simulink model "power_system"  (R2019a)
settings: Solver=FixedStepAuto  StartTime=0.0  StopTime=10.0  RelTol=1e-3
values from neighbouring files (symbols this model uses):
  numberOfBuses = 2    [init.m]
  numberOfGenerators = 4    [init.m]
undefined symbols (not defined in the file or in its folder): magnitude
libraries: simulink x8
(part 2 of 2)

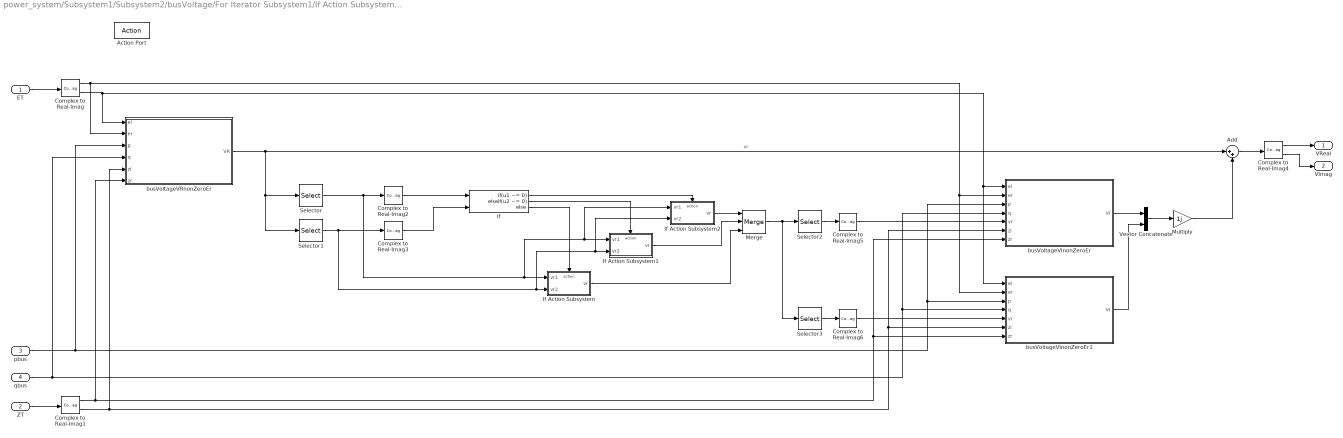
== system power_system/Subsystem1/Subsystem2/busVoltage/For Iterator Subsystem1/If Action Subsystem1/If Action Subsystem1 ==
  ET : Inport
  ZT : Inport  Port=2
  pbus : Inport  Port=3
  qbus : Inport  Port=4
  Action Port : ActionPort  ActionPortLabel=elseif(u1>u2)
  Add : Sum  Inputs=|++
  Complex to Real-Imag : ComplexToRealImag
  Complex to Real-Imag1 : ComplexToRealImag
  Complex to Real-Imag2 : ComplexToRealImag  Output=Imag
  Complex to Real-Imag3 : ComplexToRealImag  Output=Imag
  Complex to Real-Imag4 : ComplexToRealImag
  Complex to Real-Imag5 : ComplexToRealImag  Output=Real
  Complex to Real-Imag6 : ComplexToRealImag  Output=Real
  If : If  NumInputs=2  IfExpression=u1 ~= 0  ElseIfExpressions=u2 ~= 0
  If Action Subsystem : Subsystem  TreatAsAtomicUnit=on
  If Action Subsystem1 : Subsystem  TreatAsAtomicUnit=on
  If Action Subsystem2 : Subsystem  TreatAsAtomicUnit=on
  Merge : Merge  Inputs=3
  Multiply : Gain  Gain=1j
  Selector : Selector  InputPortWidth=2  IndexOptions=Index vector (dialog)  Indices=[1]  OutputSizes=1
  Selector1 : Selector  InputPortWidth=2  IndexOptions=Index vector (dialog)  Indices=[2]  OutputSizes=1
  Selector2 : Selector  InputPortWidth=2  IndexOptions=Index vector (dialog)  Indices=1  OutputSizes=1
  Selector3 : Selector  InputPortWidth=2  IndexOptions=Index vector (dialog)  Indices=2  OutputSizes=1
  Vector Concatenate : Concatenate
  busVoltageVInonZeroEr : Subsystem
  busVoltageVInonZeroEr1 : Subsystem
  busVoltageVRnonZeroEr : Subsystem
  VReal : Outport
  VImag : Outport  Port=2
  wires:
  Add/1 -> Complex to Real-Imag4/1
  Multiply/1 -> Add/2
  Vector Concatenate/1 -> Multiply/1
  busVoltageVInonZeroEr1/1(VI) -> Vector Concatenate/2
  busVoltageVInonZeroEr/1(VI) -> Vector Concatenate/1
  Complex to Real-Imag1/1 -> busVoltageVRnonZeroEr/6(zr), busVoltageVInonZeroEr1/7(zr), busVoltageVInonZeroEr/7(zr)
  Complex to Real-Imag1/2 -> busVoltageVRnonZeroEr/5(zi), busVoltageVInonZeroEr1/6(zi), busVoltageVInonZeroEr/6(zi)
  qbus/1 -> busVoltageVInonZeroEr1/4(q), busVoltageVInonZeroEr/4(q), busVoltageVRnonZeroEr/4(q)
  pbus/1 -> busVoltageVRnonZeroEr/3(p), busVoltageVInonZeroEr1/3(p), busVoltageVInonZeroEr/3(p)
  Complex to Real-Imag/1 -> busVoltageVRnonZeroEr/2(er), busVoltageVInonZeroEr1/2(er), busVoltageVInonZeroEr/2(er)
  Complex to Real-Imag/2 -> busVoltageVRnonZeroEr/1(ei), busVoltageVInonZeroEr1/1(ei), busVoltageVInonZeroEr/1(ei)
  Selector2/1 -> Complex to Real-Imag5/1
  Selector3/1 -> Complex to Real-Imag6/1
  Merge/1 -> Selector3/1, Selector2/1
  If Action Subsystem/1(vr) -> Merge/3
  If Action Subsystem1/1(vr) -> Merge/2
  If Action Subsystem2/1(vr) -> Merge/1
  Selector1/1 -> Complex to Real-Imag3/1, If Action Subsystem1/2(vr2), If Action Subsystem2/2(vr2), If Action Subsystem/2(vr2)
  If/3 -> If Action Subsystem/Action
  If/2 -> If Action Subsystem1/Action
  If/1 -> If Action Subsystem2/Action
  Complex to Real-Imag3/1 -> If/2
  Complex to Real-Imag2/1 -> If/1
  Selector/1 -> Complex to Real-Imag2/1, If Action Subsystem1/1(vr1), If Action Subsystem2/1(vr1), If Action Subsystem/1(vr1)
  busVoltageVRnonZeroEr/1(VR) -> Add/1, Selector/1, Selector1/1  "vr"
  ZT/1 -> Complex to Real-Imag1/1
  ET/1 -> Complex to Real-Imag/1
  Complex to Real-Imag4/2 -> VImag/1
  Complex to Real-Imag4/1 -> VReal/1
  Complex to Real-Imag5/1 -> busVoltageVInonZeroEr/5(vr)
  Complex to Real-Imag6/1 -> busVoltageVInonZeroEr1/5(vr)

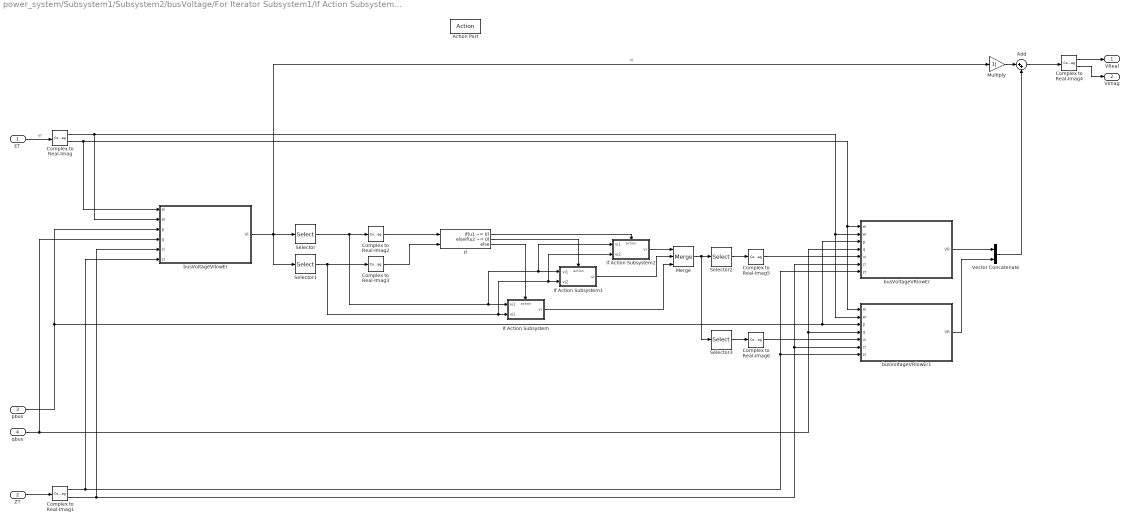
== system power_system/Subsystem1/Subsystem2/busVoltage/For Iterator Subsystem1/If Action Subsystem1/If Action Subsystem2 ==
  ET : Inport
  ZT : Inport  Port=2
  pbus : Inport  Port=3
  qbus : Inport  Port=4
  Action Port : ActionPort  ActionPortLabel=else
  Add : Sum  Inputs=|++
  Complex to Real-Imag : ComplexToRealImag
  Complex to Real-Imag1 : ComplexToRealImag
  Complex to Real-Imag2 : ComplexToRealImag  Output=Imag
  Complex to Real-Imag3 : ComplexToRealImag  Output=Imag
  Complex to Real-Imag4 : ComplexToRealImag
  Complex to Real-Imag5 : ComplexToRealImag  Output=Real
  Complex to Real-Imag6 : ComplexToRealImag  Output=Real
  If : If  NumInputs=2  IfExpression=u1 ~= 0  ElseIfExpressions=u2 ~= 0
  If Action Subsystem : Subsystem  TreatAsAtomicUnit=on
  If Action Subsystem1 : Subsystem  TreatAsAtomicUnit=on
  If Action Subsystem2 : Subsystem  TreatAsAtomicUnit=on
  Merge : Merge  Inputs=3
  Multiply : Gain  Gain=1j
  Selector : Selector  InputPortWidth=2  IndexOptions=Index vector (dialog)  Indices=[1]  OutputSizes=1
  Selector1 : Selector  InputPortWidth=2  IndexOptions=Index vector (dialog)  Indices=[2]  OutputSizes=1
  Selector2 : Selector  InputPortWidth=2  IndexOptions=Index vector (dialog)  Indices=[1]  OutputSizes=1
  Selector3 : Selector  InputPortWidth=2  IndexOptions=Index vector (dialog)  Indices=[2]  OutputSizes=1
  Vector Concatenate : Concatenate
  busVoltageVIlowEr : Subsystem
  busVoltageVRlowEr : Subsystem
  busVoltageVRlowEr1 : Subsystem
  VReal : Outport
  VImag : Outport  Port=2
  wires:
  Vector Concatenate/1 -> Add/2
  Multiply/1 -> Add/1
  Selector3/1 -> Complex to Real-Imag6/1
  Selector2/1 -> Complex to Real-Imag5/1
  ET/1 -> Complex to Real-Imag/1  "vr"
  busVoltageVRlowEr1/1(VR) -> Vector Concatenate/2
  busVoltageVRlowEr/1(VR) -> Vector Concatenate/1
  If/3 -> If Action Subsystem/Action
  Selector1/1 -> Complex to Real-Imag3/1, If Action Subsystem/2(vi2), If Action Subsystem1/2(vi2), If Action Subsystem2/2(vi2)
  If Action Subsystem1/1(vi) -> Merge/2
  If Action Subsystem2/1(vi) -> Merge/1
  Selector/1 -> Complex to Real-Imag2/1, If Action Subsystem/1(vi1), If Action Subsystem1/1(vi1), If Action Subsystem2/1(vi1)
  If Action Subsystem/1(vi) -> Merge/3
  If/2 -> If Action Subsystem1/Action
  Merge/1 -> Selector3/1, Selector2/1
  If/1 -> If Action Subsystem2/Action
  Complex to Real-Imag2/1 -> If/1
  Complex to Real-Imag3/1 -> If/2
  busVoltageVIlowEr/1(VI) -> Selector1/1, Multiply/1, Selector/1  "vi"
  qbus/1 -> busVoltageVIlowEr/4(q), busVoltageVRlowEr/4(q), busVoltageVRlowEr1/4(q)
  pbus/1 -> busVoltageVRlowEr/3(p), busVoltageVRlowEr1/3(p), busVoltageVIlowEr/3(p)
  Complex to Real-Imag/2 -> busVoltageVRlowEr/1(ei), busVoltageVRlowEr1/1(ei), busVoltageVIlowEr/1(ei)
  Complex to Real-Imag/1 -> busVoltageVRlowEr/2(er), busVoltageVRlowEr1/2(er), busVoltageVIlowEr/2(er)
  Complex to Real-Imag1/1 -> busVoltageVRlowEr/7(zr), busVoltageVRlowEr1/7(zr), busVoltageVIlowEr/6(zr)
  Complex to Real-Imag1/2 -> busVoltageVIlowEr/5(zi), busVoltageVRlowEr/6(zi), busVoltageVRlowEr1/6(zi)
  ZT/1 -> Complex to Real-Imag1/1
  Complex to Real-Imag4/1 -> VReal/1
  Complex to Real-Imag4/2 -> VImag/1
  Add/1 -> Complex to Real-Imag4/1
  Complex to Real-Imag5/1 -> busVoltageVRlowEr/5(vi)
  Complex to Real-Imag6/1 -> busVoltageVRlowEr1/5(vi)

== system power_system/Subsystem1/Subsystem2/busVoltage/For Iterator Subsystem1/If Action Subsystem1/If Action Subsystem3 ==
  Action Port : ActionPort  ActionPortLabel=if(u1 < u2)
  Constant : Constant
  v : Outport
  wires:
  Constant/1 -> v/1

== system power_system/Subsystem1/Subsystem2/busVoltage/For Iterator Subsystem1/If Action Subsystem1/If Action Subsystem4 ==
  Action Port : ActionPort  ActionPortLabel=else
  Constant : Constant  Value=2
  v : Outport
  wires:
  Constant/1 -> v/1

== system power_system/Subsystem1/Subsystem2/busVoltage/For Iterator Subsystem1/If Action Subsystem1/map to [-pi, pi] ==
  u : Inport
  Add : Sum  Inputs=||+-+
  Compare To Constant : simulink/Logic and Bit Operations/Compare To Constant  relop=>  const=pi  OutDataTypeStr=boolean
  Compare To Constant1 : simulink/Logic and Bit Operations/Compare To Constant  relop=<  const=-pi  OutDataTypeStr=boolean
  Constant : Constant  Value=2*pi
  Gain1 : Gain  Gain=2*pi
  Gain2 : Gain  Gain=2*pi
  Mod : Math  Operator=mod  SaturateOnIntegerOverflow=on
  y : Outport
  wires:
  Compare To Constant1/1 -> Gain2/1
  Compare To Constant/1 -> Gain1/1
  u/1 -> Mod/1
  Gain1/1 -> Add/2
  Mod/1 -> Compare To Constant/1, Compare To Constant1/1, Add/1
  Add/1 -> y/1
  Constant/1 -> Mod/2
  Gain2/1 -> Add/3

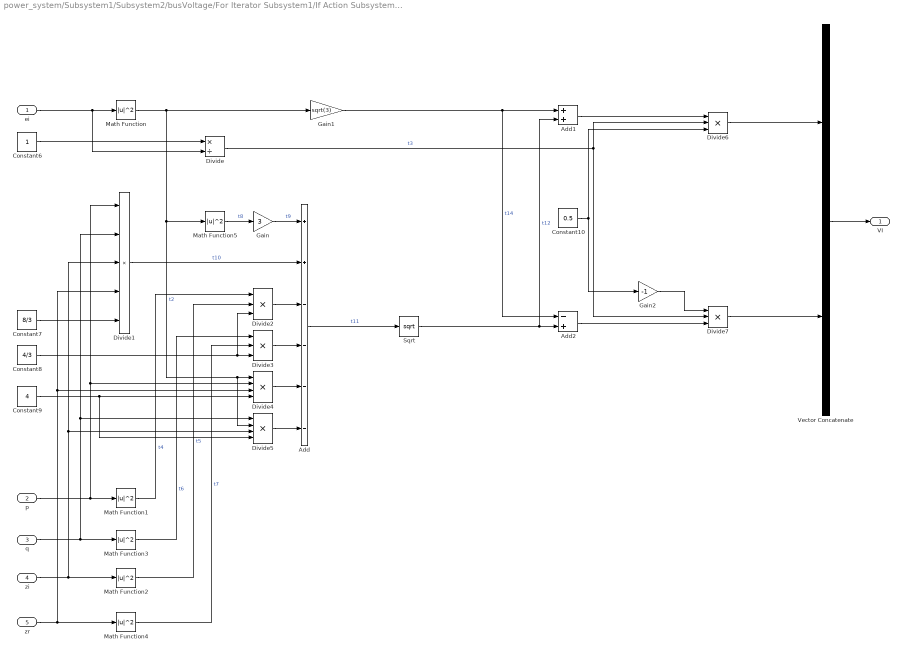
== system power_system/Subsystem1/Subsystem2/busVoltage/For Iterator Subsystem1/If Action Subsystem1/If Action Subsystem/busVoltageVIzeroEr ==
  ei : Inport
  p : Inport  Port=2
  q : Inport  Port=3
  zi : Inport  Port=4
  zr : Inport  Port=5
  Add : Sum  Inputs=++----
  Add1 : Sum
  Add2 : Sum  Inputs=-+
  Constant10 : Constant  Value=0.5
  Constant6 : Constant
  Constant7 : Constant  Value=8/3
  Constant8 : Constant  Value=4/3
  Constant9 : Constant  Value=4
  Divide : Product  Inputs=*/
  Divide1 : Product  Inputs=5
  Divide{2..3,6..7} (4 alike) : Product  Inputs=3
  Divide4 : Product  Inputs=4
  Divide5 : Product  Inputs=4
  Gain : Gain  Gain=3
  Gain1 : Gain  Gain=sqrt(3)
  Gain2 : Gain  Gain=-1
  Math Function{,1..5} (6 alike) : Math  Operator=magnitude^2  SaturateOnIntegerOverflow=on
  Sqrt : Sqrt  SaturateOnIntegerOverflow=on
  Vector Concatenate : Concatenate
  VI : Outport
  wires:
  Math Function1/1 -> Divide2/1  "t4"
  Add2/1 -> Divide7/3
  Gain2/1 -> Divide7/1
  Divide2/1 -> Add/3
  Divide1/1 -> Add/2  "t10"
  Divide6/1 -> Vector Concatenate/1
  Math Function3/1 -> Divide3/1  "t6"
  Math Function5/1 -> Gain/1  "t8"
  Constant6/1 -> Divide/1
  Add/1 -> Sqrt/1  "t11"
  Sqrt/1 -> Add2/2, Add1/2  "t12"
  zr/1 -> Math Function4/1, Divide1/4, Divide4/3
  Gain/1 -> Add/1  "t9"
  Add1/1 -> Divide6/1
  Divide/1 -> Divide7/2, Divide6/2  "t3"
  Gain1/1 -> Add1/1, Add2/1  "t14"
  Constant10/1 -> Gain2/1, Divide6/3
  p/1 -> Math Function1/1, Divide1/1, Divide4/2
  Math Function/1 -> Gain1/1, Divide4/1, Divide5/2, Math Function5/1  "t2"
  Constant9/1 -> Divide4/4, Divide5/4
  Constant8/1 -> Divide2/3, Divide3/3
  ei/1 -> Math Function/1, Divide/2
  Math Function2/1 -> Divide2/2  "t5"
  Vector Concatenate/1 -> VI/1
  Constant7/1 -> Divide1/5
  Divide7/1 -> Vector Concatenate/2
  q/1 -> Math Function3/1, Divide1/2, Divide5/1
  Divide4/1 -> Add/5
  Math Function4/1 -> Divide3/2  "t7"
  Divide5/1 -> Add/6
  zi/1 -> Math Function2/1, Divide1/3, Divide5/3
  Divide3/1 -> Add/4

== system power_system/Subsystem1/Subsystem2/busVoltage/For Iterator Subsystem1/If Action Subsystem1/If Action Subsystem/busVoltageVRzeroEr ==
  ei : Inport
  p : Inport  Port=2
  q : Inport  Port=3
  zi : Inport  Port=4
  zr : Inport  Port=5
  Add : Sum  Inputs=|+-
  Divide : Product
  Divide1 : Product
  Divide2 : Product  Inputs=/*
  Gain : Gain  Gain=sqrt(3)/3
  VR : Outport
  wires:
  Divide1/1 -> Add/1
  Divide/1 -> Add/2
  zi/1 -> Divide1/2
  Divide2/1 -> VR/1
  ei/1 -> Divide2/1
  q/1 -> Divide/1
  Add/1 -> Gain/1
  zr/1 -> Divide/2
  p/1 -> Divide1/1
  Gain/1 -> Divide2/2

== system power_system/Subsystem1/Subsystem2/busVoltage/For Iterator Subsystem1/If Action Subsystem1/If Action Subsystem1/If Action Subsystem ==
  vr1 : Inport
  vr2 : Inport  Port=2
  Action Port : ActionPort  ActionPortLabel=else
  Vector Concatenate : Concatenate
  vr : Outport
  wires:
  Vector Concatenate/1 -> vr/1
  vr2/1 -> Vector Concatenate/2
  vr1/1 -> Vector Concatenate/1

== system power_system/Subsystem1/Subsystem2/busVoltage/For Iterator Subsystem1/If Action Subsystem1/If Action Subsystem1/If Action Subsystem1 ==
  vr1 : Inport
  vr2 : Inport  Port=2
  Action Port : ActionPort  ActionPortLabel=elseif(u2 ~= 0)
  Terminator : Terminator
  Vector Concatenate : Concatenate
  vr : Outport
  wires:
  vr2/1 -> Terminator/1
  Vector Concatenate/1 -> vr/1
  vr1/1 -> Vector Concatenate/1, Vector Concatenate/2

== system power_system/Subsystem1/Subsystem2/busVoltage/For Iterator Subsystem1/If Action Subsystem1/If Action Subsystem1/If Action Subsystem2 ==
  vr1 : Inport
  vr2 : Inport  Port=2
  Action Port : ActionPort  ActionPortLabel=if(u1 ~= 0)
  Terminator : Terminator
  Vector Concatenate : Concatenate
  vr : Outport
  wires:
  vr1/1 -> Terminator/1
  Vector Concatenate/1 -> vr/1
  vr2/1 -> Vector Concatenate/2, Vector Concatenate/1

== system power_system/Subsystem1/Subsystem2/busVoltage/For Iterator Subsystem1/If Action Subsystem1/If Action Subsystem1/busVoltageVInonZeroEr ==
  ei : Inport
  er : Inport  Port=2
  p : Inport  Port=3
  q : Inport  Port=4
  vr : Inport  Port=5
  zi : Inport  Port=6
  zr : Inport  Port=7
  Add : Sum  Inputs=+-+
  Divide : Product  Inputs=*/
  Divide1 : Product  Inputs=**
  Divide2 : Product  Inputs=**
  Divide3 : Product  Inputs=**
  Gain : Gain  Gain=sqrt(3)/3
  Gain1 : Gain  Gain=sqrt(3)/3
  VI : Outport
  wires:
  Add/1 -> Divide/1
  Divide1/1 -> Add/1
  Divide3/1 -> Gain1/1
  Divide2/1 -> Gain/1
  zr/1 -> Divide3/2
  q/1 -> Divide3/1
  zi/1 -> Divide2/2
  p/1 -> Divide2/1
  vr/1 -> Divide1/2
  ei/1 -> Divide1/1
  Gain1/1 -> Add/3
  Gain/1 -> Add/2
  er/1 -> Divide/2
  Divide/1 -> VI/1

== system power_system/Subsystem1/Subsystem2/busVoltage/For Iterator Subsystem1/If Action Subsystem1/If Action Subsystem1/busVoltageVInonZeroEr1 ==
  ei : Inport
  er : Inport  Port=2
  p : Inport  Port=3
  q : Inport  Port=4
  vr : Inport  Port=5
  zi : Inport  Port=6
  zr : Inport  Port=7
  Add : Sum  Inputs=+-+
  Divide : Product  Inputs=*/
  Divide1 : Product  Inputs=**
  Divide2 : Product  Inputs=**
  Divide3 : Product  Inputs=**
  Gain : Gain  Gain=sqrt(3)/3
  Gain1 : Gain  Gain=sqrt(3)/3
  VI : Outport
  wires:
  Divide/1 -> VI/1
  er/1 -> Divide/2
  Gain/1 -> Add/2
  Gain1/1 -> Add/3
  ei/1 -> Divide1/1
  vr/1 -> Divide1/2
  p/1 -> Divide2/1
  zi/1 -> Divide2/2
  q/1 -> Divide3/1
  zr/1 -> Divide3/2
  Divide2/1 -> Gain/1
  Divide3/1 -> Gain1/1
  Divide1/1 -> Add/1
  Add/1 -> Divide/1

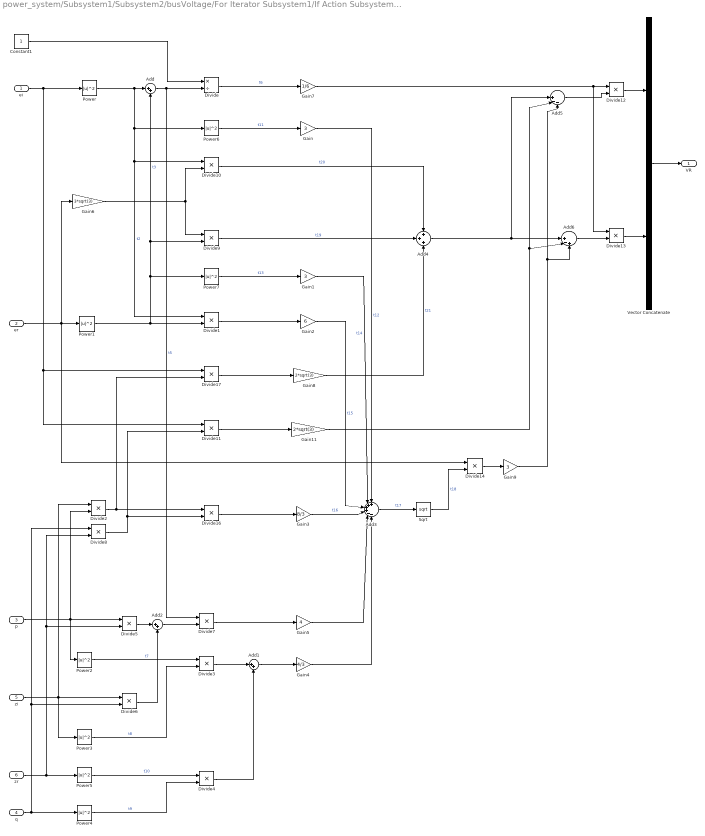
== system power_system/Subsystem1/Subsystem2/busVoltage/For Iterator Subsystem1/If Action Subsystem1/If Action Subsystem1/busVoltageVRnonZeroEr ==
  ei : Inport
  er : Inport  Port=2
  p : Inport  Port=3
  q : Inport  Port=4
  zi : Inport  Port=5
  zr : Inport  Port=6
  Add : Sum  Inputs=|++
  Add1 : Sum  Inputs=|++
  Add2 : Sum  Inputs=|++
  Add3 : Sum  Inputs=++++--
  Add4 : Sum  Inputs=+++
  Add5 : Sum  Inputs=||+--
  Add6 : Sum  Inputs=||+-+
  Constant1 : Constant
  Divide : Product  Inputs=*/
  Divide{1..14,16..17} (16 alike) : Product  Inputs=**
  Gain : Gain  Gain=3
  Gain1 : Gain  Gain=3
  Gain11 : Gain  Gain=2*sqrt(3)
  Gain2 : Gain  Gain=6
  Gain3 : Gain  Gain=8/3
  Gain4 : Gain  Gain=4/3
  Gain5 : Gain  Gain=4
  Gain6 : Gain  Gain=3*sqrt(3)
  Gain7 : Gain  Gain=1/6
  Gain8 : Gain  Gain=2*sqrt(3)
  Gain9 : Gain  Gain=3
  Power{,1..7} (8 alike) : Math  Operator=magnitude^2  SaturateOnIntegerOverflow=on
  Sqrt : Sqrt  SaturateOnIntegerOverflow=on
  Vector Concatenate : Concatenate
  VR : Outport
  wires:
  ei/1 -> Divide17/1, Divide11/1, Power/1
  Divide8/1 -> Divide16/2, Divide11/2
  Divide2/1 -> Divide16/1, Divide17/2
  zi/1 -> Power3/1, Divide2/1, Divide6/1
  zr/1 -> Power5/1, Divide8/2, Divide5/2
  q/1 -> Power4/1, Divide8/1, Divide6/2
  Divide11/1 -> Gain11/1
  Gain11/1 -> Add5/2, Add6/2
  Gain9/1 -> Add6/3, Add5/3
  Divide14/1 -> Gain9/1
  Add4/1 -> Add6/1, Add5/1
  Add6/1 -> Divide13/2
  Add5/1 -> Divide12/2
  Divide13/1 -> Vector Concatenate/2
  Divide12/1 -> Vector Concatenate/1
  Gain7/1 -> Divide12/1, Divide13/1
  Gain8/1 -> Add4/3  "t21"
  Divide17/1 -> Gain8/1
  Divide10/1 -> Add4/1  "t20"
  Divide9/1 -> Add4/2  "t19"
  Gain6/1 -> Divide10/2, Divide9/1
  er/1 -> Power1/1, Divide14/1, Gain6/1
  Sqrt/1 -> Divide14/2  "t18"
  Add3/1 -> Sqrt/1  "t17"
  Gain5/1 -> Add3/5
  Add2/1 -> Divide7/2
  Divide7/1 -> Gain5/1
  Divide6/1 -> Add2/2
  Divide5/1 -> Add2/1
  Power4/1 -> Divide4/2  "t9"
  Power5/1 -> Divide4/1  "t10"
  Gain4/1 -> Add3/6
  Add1/1 -> Gain4/1
  Divide4/1 -> Add1/2
  Divide3/1 -> Add1/1
  Gain3/1 -> Add3/4  "t16"
  Divide16/1 -> Gain3/1
  Gain2/1 -> Add3/3  "t15"
  Divide1/1 -> Gain2/1
  Gain1/1 -> Add3/2  "t14"
  Gain/1 -> Add3/1  "t12"
  Power7/1 -> Gain1/1  "t13"
  Power6/1 -> Gain/1  "t11"
  Power3/1 -> Divide3/2  "t8"
  Power2/1 -> Divide3/1  "t7"
  p/1 -> Divide2/2, Power2/1, Divide5/1
  Divide/1 -> Gain7/1  "t6"
  Constant1/1 -> Divide/1
  Add/1 -> Divide/2, Divide7/1  "t5"
  Power1/1 -> Add/2, Divide9/2, Power7/1, Divide1/2  "t3"
  Power/1 -> Divide10/1, Divide1/1, Power6/1, Add/1  "t2"
  Vector Concatenate/1 -> VR/1

== system power_system/Subsystem1/Subsystem2/busVoltage/For Iterator Subsystem1/If Action Subsystem1/If Action Subsystem2/If Action Subsystem ==
  vi1 : Inport
  vi2 : Inport  Port=2
  Action Port : ActionPort  ActionPortLabel=else
  Vector Concatenate : Concatenate
  vi : Outport
  wires:
  Vector Concatenate/1 -> vi/1
  vi2/1 -> Vector Concatenate/2
  vi1/1 -> Vector Concatenate/1

== system power_system/Subsystem1/Subsystem2/busVoltage/For Iterator Subsystem1/If Action Subsystem1/If Action Subsystem2/If Action Subsystem1 ==
  vi1 : Inport
  vi2 : Inport  Port=2
  Action Port : ActionPort  ActionPortLabel=elseif(u2 ~= 0)
  Terminator : Terminator
  Vector Concatenate : Concatenate
  vi : Outport
  wires:
  vi2/1 -> Terminator/1
  Vector Concatenate/1 -> vi/1
  vi1/1 -> Vector Concatenate/1, Vector Concatenate/2

== system power_system/Subsystem1/Subsystem2/busVoltage/For Iterator Subsystem1/If Action Subsystem1/If Action Subsystem2/If Action Subsystem2 ==
  vi1 : Inport
  vi2 : Inport  Port=2
  Action Port : ActionPort  ActionPortLabel=if(u1 ~= 0)
  Terminator : Terminator
  Vector Concatenate : Concatenate
  vi : Outport
  wires:
  vi1/1 -> Terminator/1
  Vector Concatenate/1 -> vi/1
  vi2/1 -> Vector Concatenate/2, Vector Concatenate/1

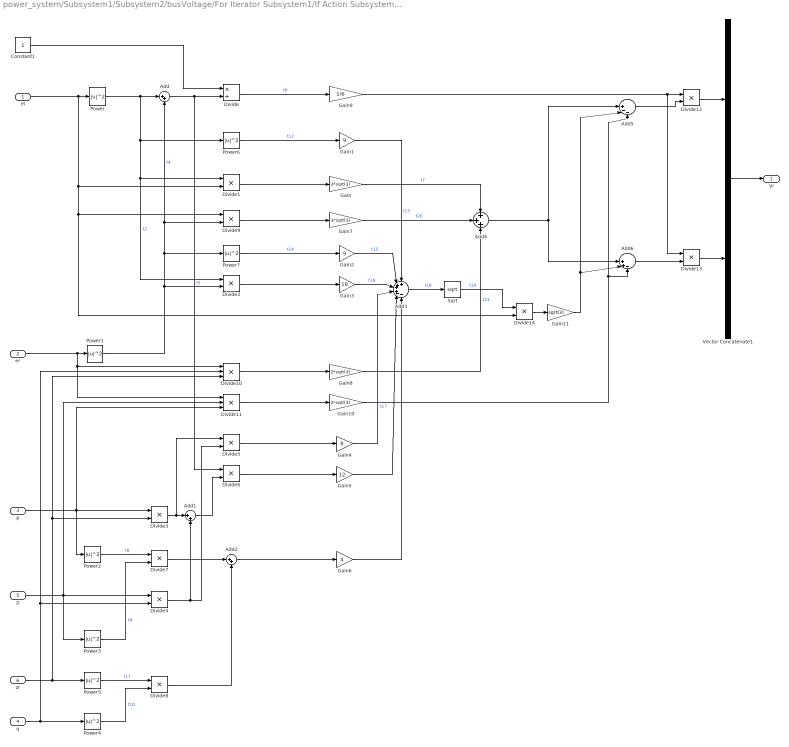
== system power_system/Subsystem1/Subsystem2/busVoltage/For Iterator Subsystem1/If Action Subsystem1/If Action Subsystem2/busVoltageVIlowEr ==
  ei : Inport
  er : Inport  Port=2
  p : Inport  Port=3
  q : Inport  Port=4
  zi : Inport  Port=5
  zr : Inport  Port=6
  Add : Sum  Inputs=|++
  Add1 : Sum  Inputs=|++
  Add2 : Sum  Inputs=|++
  Add3 : Sum  Inputs=++++--
  Add4 : Sum  Inputs=+++
  Add5 : Sum  Inputs=||+--
  Add6 : Sum  Inputs=||++-
  Constant1 : Constant
  Divide : Product  Inputs=*/
  Divide{1..2,6,9,12..14} (7 alike) : Product  Inputs=**
  Divide10 : Product  Inputs=***
  Divide11 : Product  Inputs=***
  Divide{3..5,7..8} (5 alike) : Product
  Gain : Gain  Gain=3*sqrt(3)
  Gain1 : Gain  Gain=9
  Gain10 : Gain  Gain=2*sqrt(3)
  Gain11 : Gain  Gain=sqrt(3)
  Gain2 : Gain  Gain=9
  Gain3 : Gain  Gain=18
  Gain4 : Gain  Gain=8
  Gain5 : Gain  Gain=12
  Gain6 : Gain  Gain=4
  Gain7 : Gain  Gain=3*sqrt(3)
  Gain8 : Gain  Gain=2*sqrt(3)
  Gain9 : Gain  Gain=1/6
  Power{,1..7} (8 alike) : Math  Operator=magnitude^2  SaturateOnIntegerOverflow=on
  Sqrt : Sqrt  SaturateOnIntegerOverflow=on
  Vector Concatenate1 : Concatenate
  VI : Outport
  wires:
  Gain11/1 -> Add5/2, Add6/2
  Divide14/1 -> Gain11/1
  Add4/1 -> Add5/1, Add6/1
  Gain10/1 -> Add5/3, Add6/3
  Divide11/1 -> Gain10/1
  p/1 -> Power2/1, Divide3/1, Divide11/3
  Vector Concatenate1/1 -> VI/1
  Gain9/1 -> Divide12/1, Divide13/1
  Add5/1 -> Divide12/2
  Add6/1 -> Divide13/2
  Divide13/1 -> Vector Concatenate1/2
  Divide12/1 -> Vector Concatenate1/1
  Gain8/1 -> Add4/3  "t21"
  Divide10/1 -> Gain8/1
  Gain7/1 -> Add4/2  "t20"
  Divide9/1 -> Gain7/1
  Sqrt/1 -> Divide14/1  "t19"
  Add3/1 -> Sqrt/1  "t18"
  Gain5/1 -> Add3/5
  Add2/1 -> Gain6/1
  Gain6/1 -> Add3/6
  Divide8/1 -> Add2/2
  Divide7/1 -> Add2/1
  Divide6/1 -> Gain5/1
  Add1/1 -> Divide6/2
  Gain4/1 -> Add3/4  "t17"
  Divide5/1 -> Gain4/1
  Divide4/1 -> Add1/2, Divide5/2
  Divide3/1 -> Divide5/1, Add1/1
  Gain3/1 -> Add3/3  "t16"
  Divide2/1 -> Gain3/1
  Gain2/1 -> Add3/2  "t15"
  Power7/1 -> Gain2/1  "t14"
  Gain1/1 -> Add3/1  "t13"
  Power6/1 -> Gain1/1  "t12"
  Power5/1 -> Divide8/1  "t11"
  Power4/1 -> Divide8/2  "t10"
  Power3/1 -> Divide7/2  "t9"
  Power2/1 -> Divide7/1  "t8"
  Gain/1 -> Add4/1  "t7"
  Divide1/1 -> Gain/1
  Power/1 -> Add/1, Power6/1, Divide1/1, Divide2/1  "t2"
  Power1/1 -> Divide2/2, Power7/1, Divide9/2, Add/2  "t4"
  Add/1 -> Divide/2, Divide6/1  "t5"
  Constant1/1 -> Divide/1
  Divide/1 -> Gain9/1  "t6"
  er/1 -> Power1/1, Divide10/1, Divide11/1
  q/1 -> Power4/1, Divide4/2, Divide10/2
  zr/1 -> Power5/1, Divide3/2, Divide10/3
  zi/1 -> Power3/1, Divide11/2, Divide4/1
  ei/1 -> Power/1, Divide1/2, Divide14/2, Divide9/1

== system power_system/Subsystem1/Subsystem2/busVoltage/For Iterator Subsystem1/If Action Subsystem1/If Action Subsystem2/busVoltageVRlowEr ==
  ei : Inport
  er : Inport  Port=2
  p : Inport  Port=3
  q : Inport  Port=4
  vi : Inport  Port=5
  zi : Inport  Port=6
  zr : Inport  Port=7
  Add : Sum  Inputs=++-
  Divide : Product  Inputs=*/
  Divide1 : Product  Inputs=**
  Divide2 : Product  Inputs=**
  Divide3 : Product  Inputs=**
  Gain : Gain  Gain=sqrt(3)/3
  Gain1 : Gain  Gain=sqrt(3)/3
  VR : Outport
  wires:
  Divide3/1 -> Gain1/1
  ei/1 -> Divide/2
  q/1 -> Divide3/1
  zi/1 -> Divide2/2
  vi/1 -> Divide1/2
  Divide/1 -> VR/1
  Gain/1 -> Add/2
  Gain1/1 -> Add/3
  p/1 -> Divide2/1
  zr/1 -> Divide3/2
  er/1 -> Divide1/1
  Divide2/1 -> Gain/1
  Divide1/1 -> Add/1
  Add/1 -> Divide/1

== system power_system/Subsystem1/Subsystem2/busVoltage/For Iterator Subsystem1/If Action Subsystem1/If Action Subsystem2/busVoltageVRlowEr1 ==
  ei : Inport
  er : Inport  Port=2
  p : Inport  Port=3
  q : Inport  Port=4
  vi : Inport  Port=5
  zi : Inport  Port=6
  zr : Inport  Port=7
  Add : Sum  Inputs=++-
  Divide : Product  Inputs=*/
  Divide1 : Product  Inputs=**
  Divide2 : Product  Inputs=**
  Divide3 : Product  Inputs=**
  Gain : Gain  Gain=sqrt(3)/3
  Gain1 : Gain  Gain=sqrt(3)/3
  VR : Outport
  wires:
  Add/1 -> Divide/1
  Divide1/1 -> Add/1
  Divide2/1 -> Gain/1
  er/1 -> Divide1/1
  zr/1 -> Divide3/2
  p/1 -> Divide2/1
  Gain1/1 -> Add/3
  Gain/1 -> Add/2
  Divide/1 -> VR/1
  vi/1 -> Divide1/2
  zi/1 -> Divide2/2
  q/1 -> Divide3/1
  ei/1 -> Divide/2
  Divide3/1 -> Gain1/1

== matlab function power_system/Subsystem1/MATLAB Function1 ==
  data: u input
function stopper(u)
%#codegen
if ( u < -1)
    error('Bus voltage calculations have been invalid for 1 second, stopping stimulation');
end
